simulink model "CryoDet12Chan"  (R2015b)
settings: Solver=ode45  SolverMode=SingleTasking  StartTime=0.0  StopTime=10e-4  MaxStep=1e-9  RelTol=1e-3
values from neighbouring files (symbols this model uses):
  Fclk = Fadc/2    (= 185000000)    [setupCryoFPGA.m]    (also in setupCryoNew.m)
  freqBusAddrBits = 4    [setupCryoNew.m]
  noise = ifft(exp(2i*pi*rand(1, noiseLen)) .* fft(fir1(noiseLen-1, noiseBW/Fclk*noiseSteps)))    [setupCryoFPGA.m]    (also in setupCryoNew.m = exp(2i*pi*rand(1, noiseLen)))
  noiseLen = 128    [setupCryoFPGA.m]    (also in setupCryoNew.m)
  noiseSteps = 32    [setupCryoFPGA.m]    (also in setupCryoNew.m)
  notch = tf( [1 a*wNotch/Q wNotch^2], [1 wNotch/Q wNotch^2])    [setupCryoNew.m]
  notch2 = tf( [1 a*wNotch/Q wNotch^2], [1 wNotch/Q wNotch^2])    [setupCryoNew.m]
  Tclk = 1/Fclk    (= 5.40540540541e-09)    [setupCryoFPGA.m]    (also in setupCryoNew.m)
undefined symbols (not defined in the file or in its folder): AXI4, Lite, notch3, notch4, xlipgetpartsetting
libraries: xbsIndex_r4 x1191
(part 9 of 9)

== system CryoDet12Chan/DspCore/AdcDac 0/twelveLineUDC 0/SBdemod/CIC reset ==
  note: where N is number of channels in CIC filter
  note: reset latched resetIn
  note: latch resetIn
  note: CIC reset
      |
      | Synchronizes a CIC compiler 4.0 multi-channel CIC filter
      | to input channels
      |
      | Generates:
      | 1	notResetOut to CIC aresetn
      | 2	tlast to CIC tlast input
      |
      | Inputs:
      | 1	reset in
      | 2	Channel number (0-N) which may go to sel input of mux generating the input data stream
      | 3	N-2 which tells this module how deep is the multiplexing (e.g. N-2 = 10 for a 12 channel CIC filter (sorry))
      |
      | Guarantees:
      | 1	reset out is at least 2 clocks long
      | 2	end of reset occurs 2 clocks before channel 0
      | 3	tlast comes with channel N-1
      |
      | Assumes:
      | CIC oversampling set to "Sample period" = 1
      | No "streaming interface"
  resetIn : Inport
  Channel : Inport  Port=2
  N-2 : Inport  Port=3
  Constant : xbsIndex_r4/Constant  const=0  gui_display_data_type=Boolean  arith_type=Boolean  n_bits=16  bin_pt=14  preci_type=Single  exp_width=8  frac_width=24  explicit_period=off  period=1  equ=P=C  opselect=C  inp2=PCIN>>17  opr=+  inp1=P  carry=CIN  dbl_ovrd=off  block_type=constant
  Delay1 : xbsIndex_r4/Delay  rst=off  infoeditControl=Selection of Reset will increase slice count due to use of real FFs and instead of SRLs  en=off  latency=1  reg_retiming=off  dbl_ovrd=off  block_type=delay
  Delay2 : xbsIndex_r4/Delay  rst=off  infoeditControl=Selection of Reset will increase slice count due to use of real FFs and instead of SRLs  en=off  latency=1  reg_retiming=off  dbl_ovrd=off  block_type=delay
  Delay3 : xbsIndex_r4/Delay  rst=off  infoeditControl=Selection of Reset will increase slice count due to use of real FFs and instead of SRLs  en=off  latency=1  reg_retiming=off  dbl_ovrd=off  block_type=delay
  Inverter : xbsIndex_r4/Inverter  en=off  latency=2  dbl_ovrd=off  block_type=inv
  Inverter1 : xbsIndex_r4/Inverter  en=off  latency=0  dbl_ovrd=off  block_type=inv
  Logical : xbsIndex_r4/Logical  logical_function=AND  inputs=4  en=off  latency=0  precision=User Defined  arith_type=Boolean  n_bits=1  bin_pt=0  align_bp=on  dbl_ovrd=off  block_type=logical
  Logical1 : xbsIndex_r4/Logical  logical_function=OR  inputs=2  en=off  latency=0  precision=User Defined  arith_type=Boolean  n_bits=1  bin_pt=0  align_bp=on  dbl_ovrd=off  block_type=logical
  Mux : xbsIndex_r4/Mux  inputs=2  en=off  latency=0  precision=Full  arith_type=Unsigned  n_bits=16  bin_pt=14  quantization=Truncate  overflow=Wrap  dbl_ovrd=off  block_type=mux
  Relational1 : xbsIndex_r4/Relational  mode=a=b  op_type=Bool  en=off  latency=0  dbl_ovrd=off  block_type=relational
  notResetOut : Outport
  tlast : Outport  Port=2
  wires:
  resetIn/1 -> Inverter/1, Logical1/1
  Channel/1 -> Relational1/1
  N-2/1 -> Relational1/2
  Relational1/1 -> Logical/4, Delay1/1
  Logical1/1 -> Inverter1/1, Delay2/1
  Mux/1 -> Logical1/2
  Delay2/1 -> Logical/2, Delay3/1, Mux/2
  Constant/1 -> Mux/3
  Logical/1 -> Mux/1
  Delay1/1 -> tlast/1
  Inverter/1 -> Logical/1
  Delay3/1 -> Logical/3
  Inverter1/1 -> notResetOut/1
